simulink model "Model"  (R2024b)
settings: Solver=FixedStepAuto  StartTime=0.0  StopTime=10  FixedStep=1e-5  RelTol=1e-3
undefined symbols (not defined in the file): param, x0
settings Model: Creator=Nabil  LastModifiedBy=Nabil
settings DebuggingCC: UnderSpecifiedDimensionMsg=warning
settings RTWCC: GenCodeOnly=on

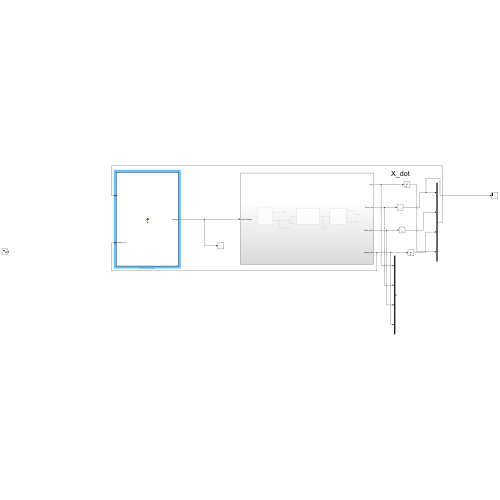
[thumbnail: Simulink's stored preview of the top-level diagram]
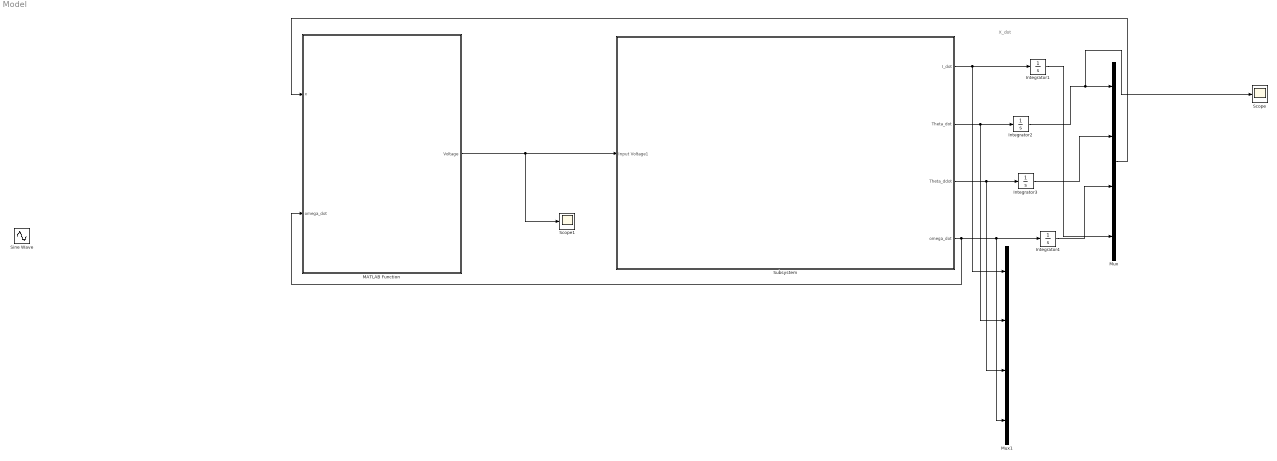
== system Model ==
  note: X_dot
  Integrator1 : Integrator  InitialCondition=x0(4)
  Integrator2 : Integrator  InitialCondition=x0(1)
  Integrator3 : Integrator  InitialCondition=x0(2)
  Integrator4 : Integrator  InitialCondition=x0(3)
  MATLAB Function : MATLAB Function  TreatAsAtomicUnit=on
  Mux : Mux
  Mux1 : Mux
  Scope : Scope
  Scope1 : Scope
  Sine Wave : Sin  Amplitude=4  Frequency=5  SampleTime=0
  Subsystem : Subsystem
  wires:
  Subsystem/2(Theta_dot) -> Mux1/2, Integrator2/1
  Subsystem/3(Theta_ddot) -> Mux1/3, Integrator3/1
  Subsystem/4(omega_dot) -> MATLAB Function/2(omega_dot), Mux1/4, Integrator4/1
  Mux/1 -> MATLAB Function/1(x)
  Subsystem/1(I_dot) -> Mux1/1, Integrator1/1
  MATLAB Function/1(Voltage) -> Scope1/1, Subsystem/1(Input Voltage1)
  Integrator2/1 -> Scope/1, Mux/1
  Integrator4/1 -> Mux/3
  Integrator3/1 -> Mux/2
  Integrator1/1 -> Mux/4

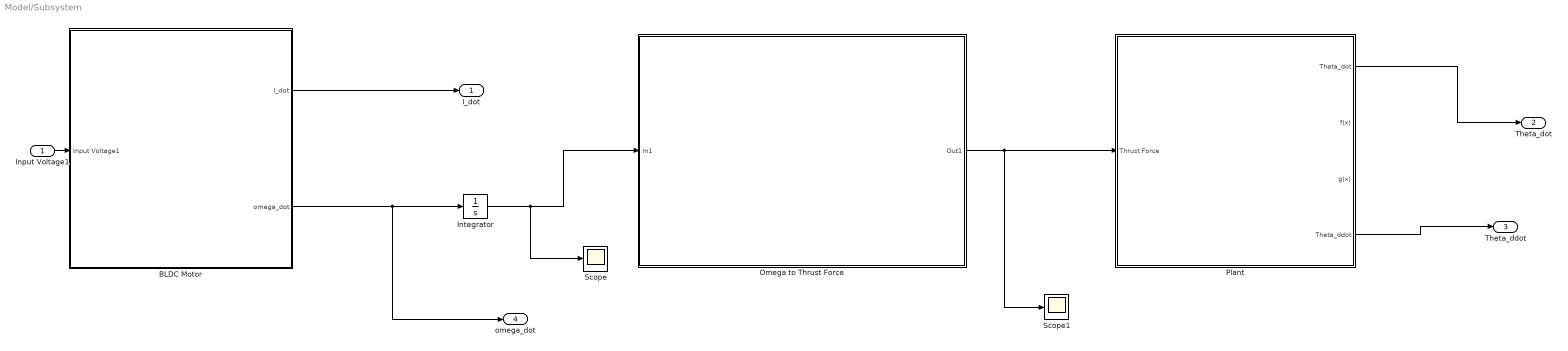
== system Model/Subsystem ==
  Input Voltage1 : Inport
  BLDC Motor : Subsystem
      mask Display: image('2200kv-brushless-motor.jpg');
  Integrator : Integrator
  Omega to Thrust Force : Subsystem
      mask Display: image('Thrust.png');
  Plant : Subsystem
      mask Display: image('1DoF.png');
  Scope : Scope
  Scope1 : Scope
  I_dot : Outport
  Theta_dot : Outport  Port=2
  Theta_ddot : Outport  Port=3
  omega_dot : Outport  Port=4
  wires:
  BLDC Motor/1(I_dot) -> I_dot/1
  BLDC Motor/2(omega_dot) -> omega_dot/1, Integrator/1
  Integrator/1 -> Scope/1, Omega to Thrust Force/1(In1)
  Omega to Thrust Force/1(Out1) -> Scope1/1, Plant/1(Thrust Force)
  Plant/4(Theta_ddot) -> Theta_ddot/1
  Plant/1(Theta_dot) -> Theta_dot/1
  Input Voltage1/1 -> BLDC Motor/1(Input Voltage1)

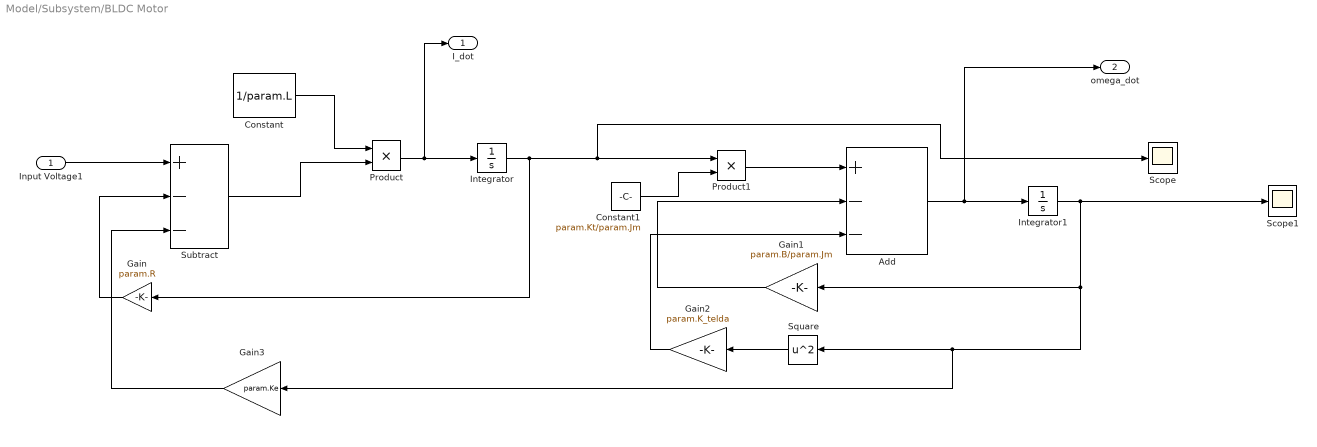
== system Model/Subsystem/BLDC Motor ==
  Input Voltage1 : Inport
  Add : Sum  Inputs=+--
  Constant : Constant  Value=1/param.L
  Constant1 : Constant  Value=param.Kt/param.Jm
  Gain : Gain  Gain=param.R
  Gain1 : Gain  Gain=param.B/param.Jm
  Gain2 : Gain  Gain=param.K_telda
  Gain3 : Gain  Gain=param.Ke
  Integrator : Integrator
  Integrator1 : Integrator
  Product : Product
  Product1 : Product
  Scope : Scope
  Scope1 : Scope
  Square : Math  Operator=square
  Subtract : Sum  Inputs=+--
  I_dot : Outport
  omega_dot : Outport  Port=2
  wires:
  Constant/1 -> Product/1
  Input Voltage1/1 -> Subtract/1
  Product/1 -> I_dot/1, Integrator/1
  Integrator/1 -> Gain/1, Scope/1, Product1/1
  Gain/1 -> Subtract/2
  Subtract/1 -> Product/2
  Constant1/1 -> Product1/2
  Product1/1 -> Add/1
  Add/1 -> omega_dot/1, Integrator1/1
  Square/1 -> Gain2/1
  Gain2/1 -> Add/3
  Gain1/1 -> Add/2
  Integrator1/1 -> Gain3/1, Square/1, Gain1/1, Scope1/1
  Gain3/1 -> Subtract/3

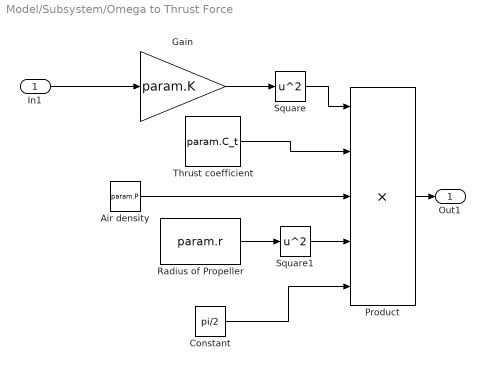
== system Model/Subsystem/Omega to Thrust Force ==
  In1 : Inport
  Air density : Constant  Value=param.P
  Constant : Constant  Value=pi/2
  Gain : Gain  Gain=param.K
  Product : Product  Inputs=5
  Radius of Propeller : Constant  Value=param.r
  Square : Math  Operator=square
  Square1 : Math  Operator=square
  Thrust coefficient : Constant  Value=param.C_t
  Out1 : Outport
  wires:
  In1/1 -> Gain/1
  Air density/1 -> Product/3
  Constant/1 -> Product/5
  Thrust coefficient/1 -> Product/2
  Square/1 -> Product/1
  Square1/1 -> Product/4
  Radius of Propeller/1 -> Square1/1
  Gain/1 -> Square/1
  Product/1 -> Out1/1

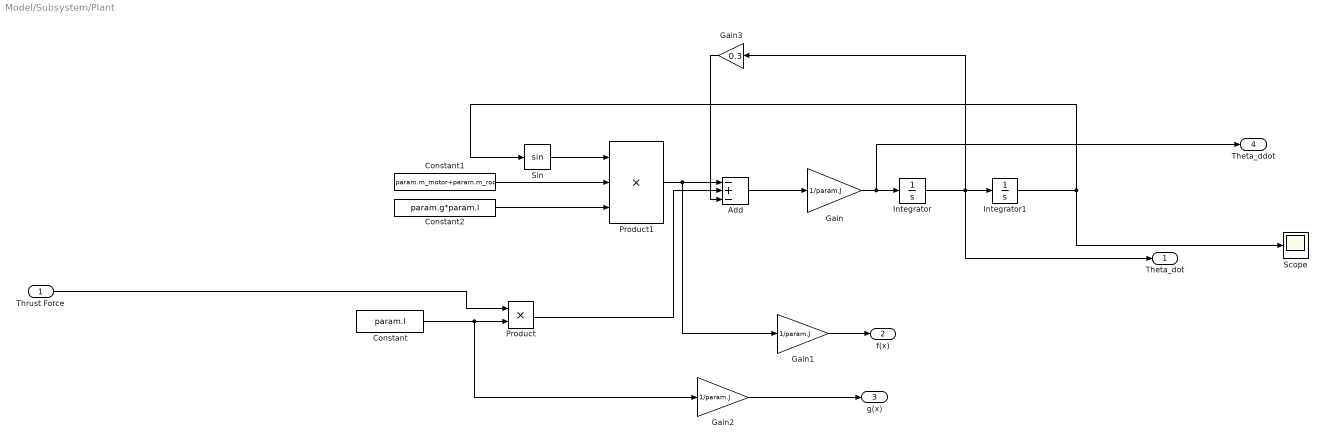
== system Model/Subsystem/Plant ==
  Thrust Force : Inport
  Add : Sum  Inputs=-+-
  Constant : Constant  Value=param.l
  Constant1 : Constant  Value=param.m_motor+param.m_rod
  Constant2 : Constant  Value=param.g*param.l
  Gain : Gain  Gain=1/param.J
  Gain1 : Gain  Gain=1/param.J
  Gain2 : Gain  Gain=1/param.J
  Gain3 : Gain  Gain=0.3
  Integrator : Integrator  InitialCondition=x0(1)
  Integrator1 : Integrator  InitialCondition=x0(2)
  Product : Product
  Product1 : Product  Inputs=3
  Scope : Scope
  Sin : Trigonometry
  Theta_dot : Outport
  f(x) : Outport  Port=2
  g(x) : Outport  Port=3
  Theta_ddot : Outport  Port=4
  wires:
  Integrator1/1 -> Sin/1, Scope/1
  Constant/1 -> Gain2/1, Product/2
  Gain/1 -> Theta_ddot/1, Integrator/1
  Integrator/1 -> Gain3/1, Theta_dot/1, Integrator1/1
  Sin/1 -> Product1/1
  Product1/1 -> Gain1/1, Add/1
  Add/1 -> Gain/1
  Constant1/1 -> Product1/2
  Constant2/1 -> Product1/3
  Product/1 -> Add/2
  Thrust Force/1 -> Product/1
  Gain1/1 -> f(x)/1
  Gain2/1 -> g(x)/1
  Gain3/1 -> Add/3

== matlab function Model/MATLAB Function ==
  data: x input; Voltage output double size=1; omega_dot input
function Voltage = fcn(x,omega_dot)
% Input-Output Linearization Control implementation for Simulink
% Inputs:
% x - State vector [theta, theta_dot, I, omega]
% omega_dot - Rotational acceleration
% theta_desired - Desired angular position
% theta_desired_dot - Desired angular velocity
% theta_desired_ddot - Desired angular acceleration

% Parameters
m_motor = 52e-3;                % Mass of motor [kg]
r_propeller = 0.15;             % Propeller radius [m]
Jm = (1/2) * m_motor * r_propeller^2; % Motor's moment of inertia

% Electrical Parameters
R = 0.09;          % Resistance (Ohms)
L = 50e-6;         % Inductance (H)
Ke = 0.00434;      % Back-EMF constant (V-s/rad)
Kt = 0.00434;      % Torque constant (Nm/A)
B = 0.001;         % Damping coefficient (Nm-s/rad)

% System Parameters
m_rod = 0.198;                   % Mass of the rod [kg]
l = 0.3;                         % Length of the rod [m]
J_rod = m_rod * l^2; % Rod's moment of inertia
m = m_rod + m_motor; % Total mass
J = J_rod + Jm;      % Total inertia
g = 9.81;                        % Gravitational acceleration [m/s^2]

% Thrust Force Parameters
K = 1.732;          % Thrust constant
K_telda = 0.1;     % Nonlinear drag coefficient

% Control Gains
% k1 = (3+m*g*l)*(J/L); 
% k2 = 9*J/l; 
% k3 = (J/Kt)*(12+K_telda/J); 
% k4 = 7*J/Kt; 
k1 = 120; 
k2 = -122; 
k3 = 49; 
k4 = 14; 


% Extract state variables
theta = x(1);
theta_dot = x(2);
I = x(3);
omega = x(4);


F = K*omega^2;
F = max(0, F);
F_dot = 2*K*omega*omega_dot;

theta_ddot = -(m*g*l/J) * sin(theta) + (l/J)*F;
theta_dddot = -(m*g*l/J) * cos(theta) * theta_dot + (l/J)*F_dot;

omega_ddot = (1/(2*K*omega))*(-2*K*omega_dot^2 + (J/L)*((m*g*l/J)*(sin(theta)*theta_dot- cos(theta)*theta_dddot)-k1*theta - k2*theta_dot-k3* theta_ddot - k4*theta_dddot));
Voltage = (J*omega_ddot + B*omega_dot + 2*K_telda*omega^2*omega_dot)*(L/Kt)+I*R + Ke* omega;
Voltage = max(0, min(22, Voltage));

end
